simulink model "new_linear"  (R2022b)
settings: Solver=VariableStepAuto  StartTime=0.0  StopTime=10.0  RelTol=1e-3
values from neighbouring files (symbols this model uses):
  e_AG = 0.2    [constantes_NoLineal.m]
  e_AN = 0.2    [constantes_NoLineal.m]
  e_GA = 1-e_AG    (= 0.8)    [constantes_NoLineal.m]
  e_GP = 0.7    [constantes_NoLineal.m]
  e_NA = 1-e_AN    (= 0.8)    [constantes_NoLineal.m]
  e_NP = 0.7    [constantes_NoLineal.m]
  pob_a = 50000    [constantes_NoLineal.m]
  pob_g = 30000    [constantes_NoLineal.m]
  pob_n = 30000    [constantes_NoLineal.m]
  pob_p = 50000    [constantes_NoLineal.m]
  rc_a = 0.003    [constantes_NoLineal.m]
  rc_g = 0.8    [constantes_NoLineal.m]
  rc_n = 0.8    [constantes_NoLineal.m]
  rc_p = 0.003    [constantes_NoLineal.m]
  scale = 1    [constantes_NoLineal.m]
  T_a = 0.2    [constantes_NoLineal.m]
  T_g = 0.7    [constantes_NoLineal.m]
  T_n = 0.7    [constantes_NoLineal.m]
  T_p = 0.2    [constantes_NoLineal.m]
settings Model: Creator=mluser  LastModifiedBy=Hoyos O

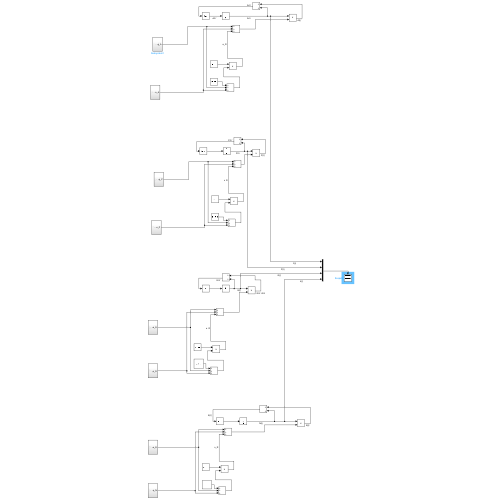
[thumbnail: Simulink's stored preview of the top-level diagram]
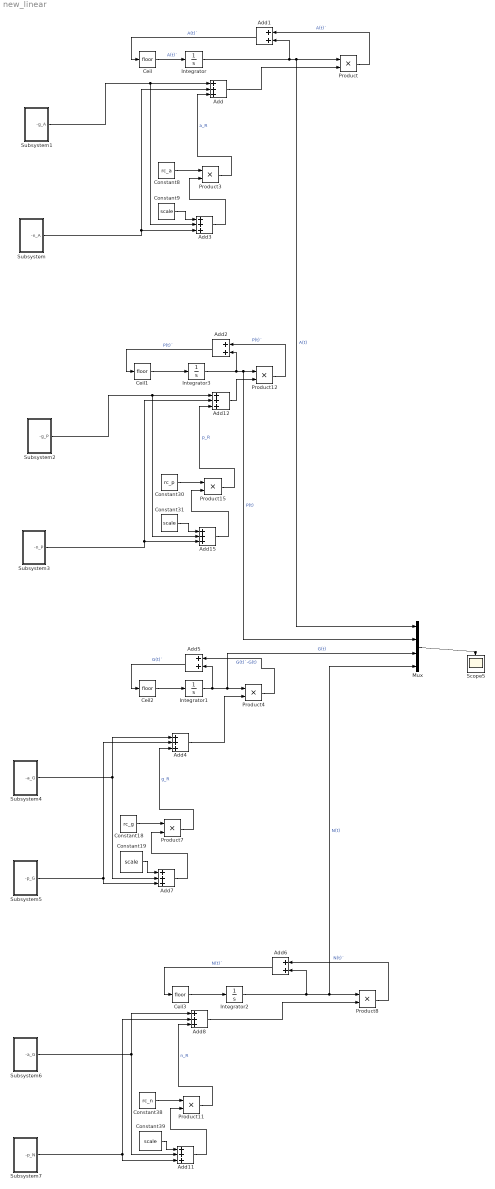
== system new_linear ==
  Add{,3..4,7..8,11..12,15} (8 alike) : Sum  Inputs=+++
  Add{1..2,5..6} (4 alike) : Sum
  Ceil{,1..3} (4 alike) : Rounding
  Constant18 : Constant  Value=rc_g
  Constant{9,19,31,39} (4 alike) : Constant  Value=scale
  Constant30 : Constant  Value=rc_p
  Constant38 : Constant  Value=rc_n
  Constant8 : Constant  Value=rc_a
  Integrator : Integrator  InitialCondition=pob_a
  Integrator1 : Integrator  InitialCondition=pob_g
  Integrator2 : Integrator  InitialCondition=pob_n
  Integrator3 : Integrator  InitialCondition=pob_p
  Mux : Mux
  Product{,3..4,7..8,11..12,15} (8 alike) : Product
  Scope5 : Scope
  Subsystem : Subsystem
  Subsystem1 : Subsystem
  Subsystem2 : Subsystem
  Subsystem3 : Subsystem
  Subsystem4 : Subsystem
  Subsystem5 : Subsystem
  Subsystem6 : Subsystem
  Subsystem7 : Subsystem
  wires:
  Integrator/1 -> Add1/2, Mux/1, Product/1  "A(t)"
  Add/1 -> Product/2
  Product3/1 -> Add/3  "a_R"
  Add3/1 -> Product3/2
  Constant8/1 -> Product3/1
  Constant9/1 -> Add3/1
  Add1/1 -> Ceil/1  "A(t)´"
  Add7/1 -> Product7/2
  Add4/1 -> Product4/2
  Integrator1/1 -> Add5/2, Mux/3, Product4/1  "G(t)"
  Add5/1 -> Ceil2/1  "G(t)´"
  Constant19/1 -> Add7/1
  Constant18/1 -> Product7/1
  Product7/1 -> Add4/3  "g_R"
  Add15/1 -> Product15/2
  Add11/1 -> Product11/2
  Add2/1 -> Ceil1/1  "P(t)´"
  Constant31/1 -> Add15/1
  Add8/1 -> Product8/2
  Integrator2/1 -> Add6/2, Mux/4, Product8/1  "N(t)"
  Constant38/1 -> Product11/1
  Product11/1 -> Add8/3  "n_R"
  Constant39/1 -> Add11/1
  Integrator3/1 -> Add2/2, Mux/2, Product12/1  "P(t)"
  Add6/1 -> Ceil3/1  "N(t)´"
  Constant30/1 -> Product15/1
  Add12/1 -> Product12/2
  Product15/1 -> Add12/3  "p_R"
  Mux/1 -> Scope5/1
  Ceil/1 -> Integrator/1  "A(t)´"
  Ceil1/1 -> Integrator3/1
  Ceil2/1 -> Integrator1/1
  Ceil3/1 -> Integrator2/1
  Subsystem/1(-n_A) -> Add3/3, Add/2
  Subsystem1/1(-g_A) -> Add3/2, Add/1
  Subsystem2/1(-g_P) -> Add15/2, Add12/1
  Subsystem3/1(-n_P) -> Add15/3, Add12/2
  Subsystem4/1(-a_G) -> Add4/1, Add7/2
  Subsystem5/1(-p_G) -> Add7/3, Add4/2
  Subsystem6/1(-a_G) -> Add11/2, Add8/1
  Subsystem7/1(-p_N) -> Add11/3, Add8/2
  Product/1 -> Add1/1  "A(t)´"
  Product12/1 -> Add2/1  "P(t)´"
  Product4/1 -> Add5/1  "G(t)´-G(t)"
  Product8/1 -> Add6/1  "N(t)´"

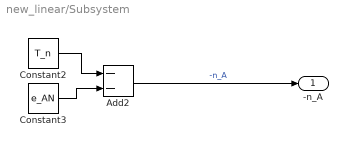
== system new_linear/Subsystem ==
  Add2 : Sum  Inputs=--
  Constant2 : Constant  Value=T_n
  Constant3 : Constant  Value=e_AN
  -n_A : Outport
  wires:
  Constant2/1 -> Add2/1
  Add2/1 -> -n_A/1  "-n_A"
  Constant3/1 -> Add2/2

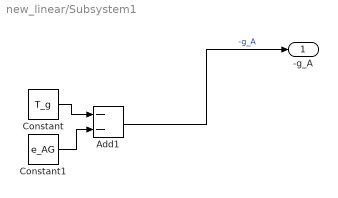
== system new_linear/Subsystem1 ==
  Add1 : Sum  Inputs=--
  Constant : Constant  Value=T_g
  Constant1 : Constant  Value=e_AG
  -g_A : Outport
  wires:
  Constant1/1 -> Add1/2
  Constant/1 -> Add1/1
  Add1/1 -> -g_A/1  "-g_A"

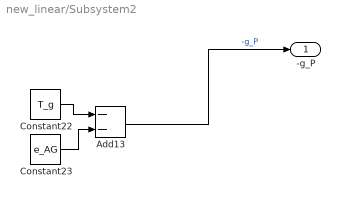
== system new_linear/Subsystem2 ==
  Add13 : Sum  Inputs=--
  Constant22 : Constant  Value=T_g
  Constant23 : Constant  Value=e_AG
  -g_P : Outport
  wires:
  Constant22/1 -> Add13/1
  Constant23/1 -> Add13/2
  Add13/1 -> -g_P/1  "-g_P"

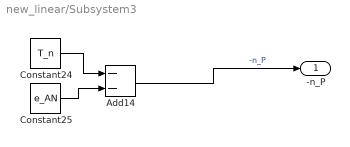
== system new_linear/Subsystem3 ==
  Add14 : Sum  Inputs=--
  Constant24 : Constant  Value=T_n
  Constant25 : Constant  Value=e_AN
  -n_P : Outport
  wires:
  Constant25/1 -> Add14/2
  Constant24/1 -> Add14/1
  Add14/1 -> -n_P/1  "-n_P"

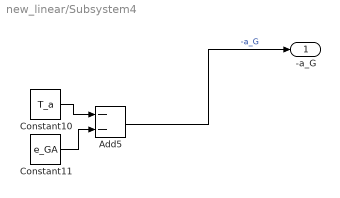
== system new_linear/Subsystem4 ==
  Add5 : Sum  Inputs=--
  Constant10 : Constant  Value=T_a
  Constant11 : Constant  Value=e_GA
  -a_G : Outport
  wires:
  Constant10/1 -> Add5/1
  Constant11/1 -> Add5/2
  Add5/1 -> -a_G/1  "-a_G"

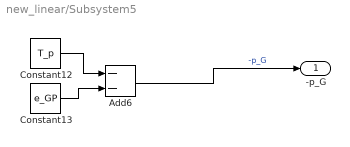
== system new_linear/Subsystem5 ==
  Add6 : Sum  Inputs=--
  Constant12 : Constant  Value=T_p
  Constant13 : Constant  Value=e_GP
  -p_G : Outport
  wires:
  Constant13/1 -> Add6/2
  Constant12/1 -> Add6/1
  Add6/1 -> -p_G/1  "-p_G"

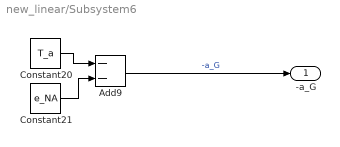
== system new_linear/Subsystem6 ==
  Add9 : Sum  Inputs=--
  Constant20 : Constant  Value=T_a
  Constant21 : Constant  Value=e_NA
  -a_G : Outport
  wires:
  Constant21/1 -> Add9/2
  Constant20/1 -> Add9/1
  Add9/1 -> -a_G/1  "-a_G"

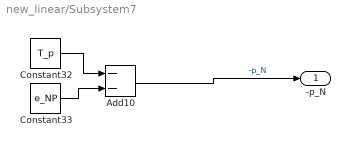
== system new_linear/Subsystem7 ==
  Add10 : Sum  Inputs=--
  Constant32 : Constant  Value=T_p
  Constant33 : Constant  Value=e_NP
  -p_N : Outport
  wires:
  Constant32/1 -> Add10/1
  Constant33/1 -> Add10/2
  Add10/1 -> -p_N/1  "-p_N"
